simulink model "Model_3"  (R2017b)
settings: Solver=ode45  StartTime=0.0  StopTime=0.01  MaxStep=1e-6  RelTol=1e-3
settings Model: Creator=lukasschwoerer  LastModifiedBy=lukasschwoerer

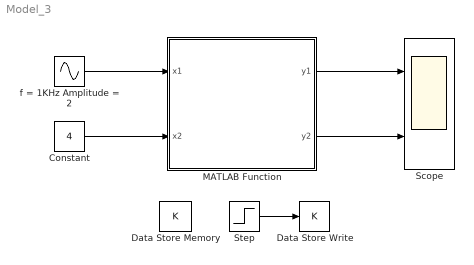
== system Model_3 ==
  Constant : Constant  Value=4
  Data Store Memory : DataStoreMemory  DataStoreName=K  ReadBeforeWriteMsg=warning  WriteAfterWriteMsg=warning  WriteAfterReadMsg=warning  ShowAdditionalParam=off  OutDataTypeStr=double
  Data Store Write : DataStoreWrite  DataStoreName=K
  MATLAB Function : MATLAB Function  TreatAsAtomicUnit=on
  Scope : Scope  NumInputPorts=2
  Step : Step  Time=0.005  After=10  SampleTime=0
  f = 1KHz Amplitude = 2 : Sin  Amplitude=2  Frequency=2*pi*1e3  SampleTime=0
  wires:
  f = 1KHz Amplitude = 2/1 -> MATLAB Function/1(x1)
  Constant/1 -> MATLAB Function/2(x2)
  MATLAB Function/1(y1) -> Scope/1
  MATLAB Function/2(y2) -> Scope/2
  Step/1 -> Data Store Write/1

== matlab function Model_3/MATLAB Function ==
  data: x1 input; y1 output; x2 input; y2 output; K data_store_memory
function [y1,y2] = kennlinie(x1,x2)

% Lokale Variable
y1max = 1;

% Globale Variable
% persistent oder global
global K 

% 1. Ausgang
if(x1>1)
    y1 = y1max;    
elseif(x1<-1)
    y1 = -y1max;    
else
    y1=x1;    
end

% 2. Ausgang
y2 = K*x1*x2;
end
